simulink model "gm_Copy_of_uz_pmsm_model_9ph_21b_all_double_vnl"  (R2022a)
settings: Solver=FixedStepAuto  StartTime=0.0  StopTime=0.8  RelTol=1e-3
PreLoadFcn:
  | uz_pmsm_model_9ph_init_parameter
undefined symbols (not defined in the file or in its folder): a, b, c, friction_coefficient, inertia, k_i_d, k_i_q, k_p_d, k_p_q, Kpd, L_d, L_o1, L_o2, L_q, L_x1, L_x2, L_y1, L_y2, L_zero, polepair, psi_pm, R_1, static_friction_torque, Tnd, ts
libraries: hdlsllib x91, hdlmdlgenlib x21, simulink x18, slpidlib x2, spsAlphaBetaZerotodq0Lib x1, pid_lib x1, spsdq0toAlphaBetaZeroLib x1
(part 3 of 4)

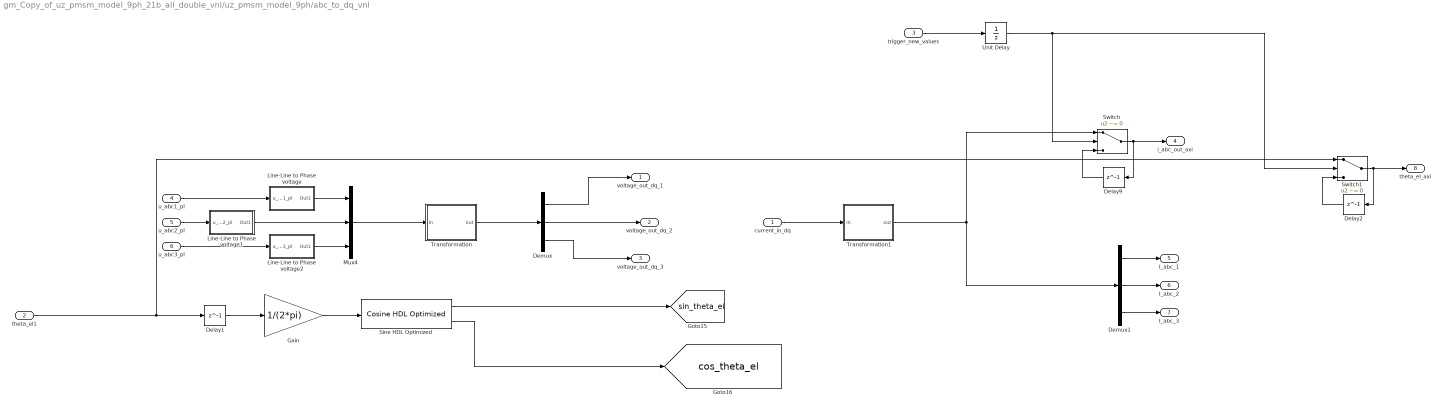
== system gm_Copy_of_uz_pmsm_model_9ph_21b_all_double_vnl/uz_pmsm_model_9ph/abc_to_dq_vnl ==
  current_in_dq : Inport
  theta_el1 : Inport  Port=2
  trigger_new_values : Inport  Port=3
  u_abc1_pl : Inport  Port=4
  u_abc2_pl : Inport  Port=5
  u_abc3_pl : Inport  Port=6
  Delay1 : Delay  DelayLength=1
  Delay2 : Delay  DelayLength=1
  Delay9 : Delay  DelayLength=1
  Demux : Demux  Outputs=3
  Demux1 : Demux  Outputs=3
  Gain : Gain  Gain=1/(2*pi)  OutDataTypeStr=fixdt(1,18,16)
  Line-Line to Phase voltage : Subsystem
  Line-Line to Phase voltage1 : Subsystem
  Line-Line to Phase voltage2 : Subsystem
  Mux4 : Mux  Inputs=3
  Sine HDL Optimized : hdlsllib/Lookup Tables/Cosine HDL Optimized  OutputFormula=sin(2*pi*u) and cos(2*pi*u)  NumDataPoints=64  TableDataTypeStr=fixdt(0,16,15)  SimulateLUTROMDelay=off
      settings: SourceProductBaseCode=SL
  Switch : Switch  Criteria=u2 ~= 0  SaturateOnIntegerOverflow=off  InputSameDT=off
  Switch1 : Switch  Criteria=u2 ~= 0  SaturateOnIntegerOverflow=off  InputSameDT=off
  Transformation : Subsystem
  Transformation1 : Subsystem
  Unit Delay : UnitDelay  SampleTime=-1  HasFrameUpgradeWarning=on
  voltage_out_dq_1 : Outport
  voltage_out_dq_2 : Outport  Port=2
  voltage_out_dq_3 : Outport  Port=3
  i_abc_out_axi : Outport  Port=4
  I_abc_1 : Outport  Port=5
  I_abc_2 : Outport  Port=6
  I_abc_3 : Outport  Port=7
  theta_el_axi : Outport  Port=8
  tag scope: cos_theta_el=global, sin_theta_el=global
  wires:
  Unit Delay/1 -> Switch/2, Switch1/2
  Switch1/1 -> Delay2/1, theta_el_axi/1
  Delay2/1 -> Switch1/3
  theta_el1/1 -> Switch1/1, Delay1/1
  Sine HDL Optimized/2 -> [cos_theta_el]
  Sine HDL Optimized/1 -> [sin_theta_el]
  Demux/3 -> voltage_out_dq_3/1
  Demux/2 -> voltage_out_dq_2/1
  Demux/1 -> voltage_out_dq_1/1
  Gain/1 -> Sine HDL Optimized/1
  u_abc1_pl/1 -> Line-Line to Phase voltage/1(u_abc1_pl)
  current_in_dq/1 -> Transformation1/1(in)
  Transformation/1(out) -> Demux/1
  Delay1/1 -> Gain/1
  Demux1/3 -> I_abc_3/1
  Switch/1 -> Delay9/1, i_abc_out_axi/1
  Demux1/1 -> I_abc_1/1
  u_abc3_pl/1 -> Line-Line to Phase voltage2/1(u_abc3_pl)
  trigger_new_values/1 -> Unit Delay/1
  Demux1/2 -> I_abc_2/1
  Mux4/1 -> Transformation/1(in)
  Delay9/1 -> Switch/3
  Line-Line to Phase voltage1/1(Out1) -> Mux4/2
  u_abc2_pl/1 -> Line-Line to Phase voltage1/1(u_abc2_pl)
  Line-Line to Phase voltage2/1(Out1) -> Mux4/3
  Line-Line to Phase voltage/1(Out1) -> Mux4/1
  Transformation1/1(out) -> Demux1/1, Switch/1

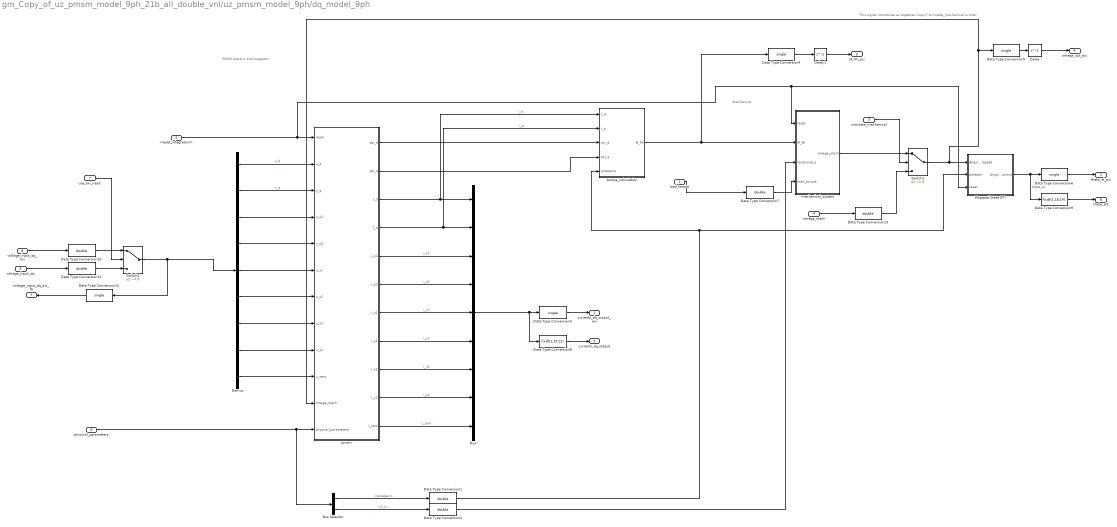
== system gm_Copy_of_uz_pmsm_model_9ph_21b_all_double_vnl/uz_pmsm_model_9ph/dq_model_9ph ==
  note: Mechanical
  note: PMSM electric and magentic
  note: This signal introduces an algebraic loop if simulate_mechanical is true!
  load_torque : Inport
  <reset_integrators> : Inport  Port=2
  simulate_mechanical : Inport  Port=3
  omega_mech : Inport  Port=4
  voltage_input_dq : Inport  Port=5
  physical_parameters : Inport  Port=6
  use_axi_input : Inport  Port=7
  voltage_input_dq_axi : Inport  Port=8
  Bus Selector : BusSelector  OutputSignals=polepair,1_J
  Data Type Conversion{1..2,7,10..11,13} (6 alike) : DataTypeConversion  OutDataTypeStr=double  RndMeth=Nearest  SaturateOnIntegerOverflow=off
  Data Type Conversion{3..6,12} (5 alike) : DataTypeConversion  OutDataTypeStr=single  RndMeth=Nearest  SaturateOnIntegerOverflow=off
  Data Type Conversion8 : DataTypeConversion  OutDataTypeStr=fixdt(1,25,12)  RndMeth=Nearest  SaturateOnIntegerOverflow=off
  Data Type Conversion9 : DataTypeConversion  OutDataTypeStr=fixdt(1,18,14)  RndMeth=Nearest  SaturateOnIntegerOverflow=off
  Delay : Delay  DelayLength=1
  Delay1 : Delay  DelayLength=1
  Demux : Demux  Outputs=9
  Mux : Mux  Inputs=9
  Switch1 : Switch  Criteria=u2 ~= 0  SaturateOnIntegerOverflow=off  InputSameDT=off
  Switch2 : Switch  Criteria=u2 ~= 0  SaturateOnIntegerOverflow=off  InputSameDT=off
  Wrapped State DTI : Subsystem
  mechanical_system : Subsystem
  pmsm : Subsystem
  torque_calculation : Subsystem
  currents_dq_output_axi : Outport
  theta_el_axi : Outport  Port=2
  M_Mi_axi : Outport  Port=3
  omega_out_axi : Outport  Port=4
  currents_dq_output : Outport  Port=5
  theta_el1 : Outport  Port=6
  voltage_input_dq_axi_fb : Outport  Port=7
  wires:
  Data Type Conversion13/1 -> Switch1/3
  Data Type Conversion12/1 -> voltage_input_dq_axi_fb/1
  Data Type Conversion11/1 -> Switch2/3
  Data Type Conversion10/1 -> Switch2/1
  voltage_input_dq_axi/1 -> Data Type Conversion10/1
  voltage_input_dq/1 -> Data Type Conversion11/1
  use_axi_input/1 -> Switch2/2
  Data Type Conversion9/1 -> theta_el1/1
  Data Type Conversion8/1 -> currents_dq_output/1
  Data Type Conversion7/1 -> mechanical_system/4(load_torque)
  Wrapped State DTI/1(Angular Position) -> Data Type Conversion6/1, Data Type Conversion9/1  "theta_el"
  Data Type Conversion6/1 -> theta_el_axi/1
  Data Type Conversion5/1 -> Delay/1
  Data Type Conversion4/1 -> Delay1/1
  Data Type Conversion3/1 -> currents_dq_output_axi/1
  Data Type Conversion2/1 -> mechanical_system/3(reciprocal_J)
  Data Type Conversion1/1 -> Wrapped State DTI/2(polepair), torque_calculation/5(polepairs)
  physical_parameters/1 -> pmsm/12(physical_parameters), Bus Selector/1
  Switch2/1 -> Demux/1, Data Type Conversion12/1
  Delay1/1 -> M_Mi_axi/1
  Delay/1 -> omega_out_axi/1
  Bus Selector/2 -> Data Type Conversion2/1  "<1_J>"
  Bus Selector/1 -> Data Type Conversion1/1  "<polepair>"
  Mux/1 -> Data Type Conversion3/1, Data Type Conversion8/1
  pmsm/8(i_y1) -> Mux/6  "i_y1"
  Switch1/1 -> Wrapped State DTI/1(Angular Speed), Data Type Conversion5/1, pmsm/11(omega_mech)
  load_torque/1 -> Data Type Conversion7/1
  mechanical_system/1(omega_mech) -> Switch1/1
  pmsm/4(I_q) -> Mux/2, torque_calculation/2(I_q)  "i_q"
  <reset_integrators>/1 -> pmsm/1(reset), mechanical_system/1(reset), Wrapped State DTI/3(reset)
  pmsm/5(i_o1) -> Mux/3  "i_o1"
  Demux/6 -> pmsm/7(u_y1)
  simulate_mechanical/1 -> Switch1/2
  pmsm/2(psi_q) -> torque_calculation/4(psi_q)
  omega_mech/1 -> Data Type Conversion13/1
  pmsm/1(psi_d) -> torque_calculation/3(psi_d)
  Demux/8 -> pmsm/9(u_y2)
  torque_calculation/1(M_Mi) -> mechanical_system/2(M_Mi), Data Type Conversion4/1
  pmsm/10(i_y2) -> Mux/8  "i_y2"
  pmsm/7(i_x1) -> Mux/5  "i_x1"
  pmsm/9(i_x2) -> Mux/7  "i_x2"
  Demux/9 -> pmsm/10(u_zero)
  Demux/2 -> pmsm/3(u_q)  "u_q"
  Demux/4 -> pmsm/5(u_o2)
  pmsm/6(i_o2) -> Mux/4  "i_o2"
  pmsm/11(i_zero) -> Mux/9  "i_zero"
  Demux/1 -> pmsm/2(u_d)  "u_d"
  pmsm/3(I_d) -> Mux/1, torque_calculation/1(I_d)  "i_d"
  Demux/3 -> pmsm/4(u_o1)
  Demux/7 -> pmsm/8(u_x2)
  Demux/5 -> pmsm/6(u_x1)

== system gm_Copy_of_uz_pmsm_model_9ph_21b_all_double_vnl/uz_pmsm_model_9ph/Compare/Assert_I_abc_1 ==
  cosim : Inport
  dut : Inport  Port=2
  AssertEq : Assertion  StopWhenAssertionFail=off
  Compare To Zero : simulink/Logic and Bit Operations/Compare To Zero  relop===  OutDataTypeStr=boolean
  Constant1 : Constant  Value=0  OutDataTypeStr=Inherit: Inherit via back propagation  SampleTime=-1
  Counter : simulink/Sources/Counter Free-Running  NumBits=32  tsamp=-1
  IgnoreCycles : Constant  Value=37  OutDataTypeStr=Inherit: Inherit via back propagation  SampleTime=-1
  Relational Operator : RelationalOperator  Operator=<  OutDataTypeStr=boolean  InputSameDT=off
  Relational Operator1 : RelationalOperator  Operator===  OutDataTypeStr=boolean  InputSameDT=off
  Switch : Switch  Criteria=u2 ~= 0  SaturateOnIntegerOverflow=off  InputSameDT=off
  Switch1 : Switch  Criteria=u2 ~= 0  SaturateOnIntegerOverflow=off  InputSameDT=off
  compare: I_abc_1 : Scope  NumInputPorts=3
  wires:
  Compare To Zero/1 -> compare: I_abc_1/3
  Relational Operator1/1 -> Compare To Zero/1, AssertEq/1  "err"
  Switch1/1 -> compare: I_abc_1/1, Relational Operator1/1
  Switch/1 -> compare: I_abc_1/2, Relational Operator1/2
  Constant1/1 -> Switch/1, Switch1/1
  Relational Operator/1 -> Switch/2, Switch1/2
  cosim/1 -> Switch1/3  "cosim"
  dut/1 -> Switch/3  "dut ref"
  Counter/1 -> Relational Operator/1
  IgnoreCycles/1 -> Relational Operator/2

== system gm_Copy_of_uz_pmsm_model_9ph_21b_all_double_vnl/uz_pmsm_model_9ph/Compare/Assert_I_abc_2 ==
  cosim : Inport
  dut : Inport  Port=2
  AssertEq : Assertion  StopWhenAssertionFail=off
  Compare To Zero : simulink/Logic and Bit Operations/Compare To Zero  relop===  OutDataTypeStr=boolean
  Constant1 : Constant  Value=0  OutDataTypeStr=Inherit: Inherit via back propagation  SampleTime=-1
  Counter : simulink/Sources/Counter Free-Running  NumBits=32  tsamp=-1
  IgnoreCycles : Constant  Value=37  OutDataTypeStr=Inherit: Inherit via back propagation  SampleTime=-1
  Relational Operator : RelationalOperator  Operator=<  OutDataTypeStr=boolean  InputSameDT=off
  Relational Operator1 : RelationalOperator  Operator===  OutDataTypeStr=boolean  InputSameDT=off
  Switch : Switch  Criteria=u2 ~= 0  SaturateOnIntegerOverflow=off  InputSameDT=off
  Switch1 : Switch  Criteria=u2 ~= 0  SaturateOnIntegerOverflow=off  InputSameDT=off
  compare: I_abc_2 : Scope  NumInputPorts=3
  wires:
  Compare To Zero/1 -> compare: I_abc_2/3
  Relational Operator1/1 -> Compare To Zero/1, AssertEq/1  "err"
  Switch1/1 -> compare: I_abc_2/1, Relational Operator1/1
  Switch/1 -> compare: I_abc_2/2, Relational Operator1/2
  Constant1/1 -> Switch/1, Switch1/1
  Relational Operator/1 -> Switch/2, Switch1/2
  cosim/1 -> Switch1/3  "cosim"
  dut/1 -> Switch/3  "dut ref"
  Counter/1 -> Relational Operator/1
  IgnoreCycles/1 -> Relational Operator/2

== system gm_Copy_of_uz_pmsm_model_9ph_21b_all_double_vnl/uz_pmsm_model_9ph/Compare/Assert_I_abc_3 ==
  cosim : Inport
  dut : Inport  Port=2
  AssertEq : Assertion  StopWhenAssertionFail=off
  Compare To Zero : simulink/Logic and Bit Operations/Compare To Zero  relop===  OutDataTypeStr=boolean
  Constant1 : Constant  Value=0  OutDataTypeStr=Inherit: Inherit via back propagation  SampleTime=-1
  Counter : simulink/Sources/Counter Free-Running  NumBits=32  tsamp=-1
  IgnoreCycles : Constant  Value=37  OutDataTypeStr=Inherit: Inherit via back propagation  SampleTime=-1
  Relational Operator : RelationalOperator  Operator=<  OutDataTypeStr=boolean  InputSameDT=off
  Relational Operator1 : RelationalOperator  Operator===  OutDataTypeStr=boolean  InputSameDT=off
  Switch : Switch  Criteria=u2 ~= 0  SaturateOnIntegerOverflow=off  InputSameDT=off
  Switch1 : Switch  Criteria=u2 ~= 0  SaturateOnIntegerOverflow=off  InputSameDT=off
  compare: I_abc_3 : Scope  NumInputPorts=3
  wires:
  Compare To Zero/1 -> compare: I_abc_3/3
  Relational Operator1/1 -> Compare To Zero/1, AssertEq/1  "err"
  Switch1/1 -> compare: I_abc_3/1, Relational Operator1/1
  Switch/1 -> compare: I_abc_3/2, Relational Operator1/2
  Constant1/1 -> Switch/1, Switch1/1
  Relational Operator/1 -> Switch/2, Switch1/2
  cosim/1 -> Switch1/3  "cosim"
  dut/1 -> Switch/3  "dut ref"
  Counter/1 -> Relational Operator/1
  IgnoreCycles/1 -> Relational Operator/2

== system gm_Copy_of_uz_pmsm_model_9ph_21b_all_double_vnl/uz_pmsm_model_9ph/Compare/Assert_i_abc_out_axi ==
  cosim : Inport
  dut : Inport  Port=2
  AssertEq : Assertion  StopWhenAssertionFail=off
  Compare To Zero : simulink/Logic and Bit Operations/Compare To Zero  relop===  OutDataTypeStr=boolean
  Constant1 : Constant  Value=0  OutDataTypeStr=Inherit: Inherit via back propagation  SampleTime=-1
  Counter : simulink/Sources/Counter Free-Running  NumBits=32  tsamp=-1
  IgnoreCycles : Constant  Value=37  OutDataTypeStr=Inherit: Inherit via back propagation  SampleTime=-1
  Relational Operator : RelationalOperator  Operator=<  OutDataTypeStr=boolean  InputSameDT=off
  Relational Operator1 : RelationalOperator  Operator===  OutDataTypeStr=boolean  InputSameDT=off
  Switch : Switch  Criteria=u2 ~= 0  SaturateOnIntegerOverflow=off  InputSameDT=off
  Switch1 : Switch  Criteria=u2 ~= 0  SaturateOnIntegerOverflow=off  InputSameDT=off
  compare: i_abc_out_axi : Scope  NumInputPorts=3
  wires:
  Compare To Zero/1 -> compare: i_abc_out_axi/3
  Relational Operator1/1 -> Compare To Zero/1, AssertEq/1  "err"
  Switch1/1 -> compare: i_abc_out_axi/1, Relational Operator1/1
  Switch/1 -> compare: i_abc_out_axi/2, Relational Operator1/2
  Constant1/1 -> Switch/1, Switch1/1
  Relational Operator/1 -> Switch/2, Switch1/2
  cosim/1 -> Switch1/3  "cosim"
  dut/1 -> Switch/3  "dut ref"
  Counter/1 -> Relational Operator/1
  IgnoreCycles/1 -> Relational Operator/2

== system gm_Copy_of_uz_pmsm_model_9ph_21b_all_double_vnl/uz_pmsm_model_9ph/Compare/Assert_theta_el_axi ==
  cosim : Inport
  dut : Inport  Port=2
  AssertEq : Assertion  StopWhenAssertionFail=off
  Compare To Zero : simulink/Logic and Bit Operations/Compare To Zero  relop===  OutDataTypeStr=boolean
  Constant1 : Constant  Value=0  OutDataTypeStr=Inherit: Inherit via back propagation  SampleTime=-1
  Counter : simulink/Sources/Counter Free-Running  NumBits=32  tsamp=-1
  IgnoreCycles : Constant  Value=37  OutDataTypeStr=Inherit: Inherit via back propagation  SampleTime=-1
  Relational Operator : RelationalOperator  Operator=<  OutDataTypeStr=boolean  InputSameDT=off
  Relational Operator1 : RelationalOperator  Operator===  OutDataTypeStr=boolean  InputSameDT=off
  Switch : Switch  Criteria=u2 ~= 0  SaturateOnIntegerOverflow=off  InputSameDT=off
  Switch1 : Switch  Criteria=u2 ~= 0  SaturateOnIntegerOverflow=off  InputSameDT=off
  compare: theta_el_axi : Scope  NumInputPorts=3
  wires:
  Compare To Zero/1 -> compare: theta_el_axi/3
  Relational Operator1/1 -> Compare To Zero/1, AssertEq/1  "err"
  Switch1/1 -> compare: theta_el_axi/1, Relational Operator1/1
  Switch/1 -> compare: theta_el_axi/2, Relational Operator1/2
  Constant1/1 -> Switch/1, Switch1/1
  Relational Operator/1 -> Switch/2, Switch1/2
  cosim/1 -> Switch1/3  "cosim"
  dut/1 -> Switch/3  "dut ref"
  Counter/1 -> Relational Operator/1
  IgnoreCycles/1 -> Relational Operator/2

== system gm_Copy_of_uz_pmsm_model_9ph_21b_all_double_vnl/uz_pmsm_model_9ph/Compare/Assert_voltage_out_dq_1 ==
  cosim : Inport
  dut : Inport  Port=2
  AssertEq : Assertion  StopWhenAssertionFail=off
  Compare To Zero : simulink/Logic and Bit Operations/Compare To Zero  relop===  OutDataTypeStr=boolean
  Constant1 : Constant  Value=0  OutDataTypeStr=Inherit: Inherit via back propagation  SampleTime=-1
  Counter : simulink/Sources/Counter Free-Running  NumBits=32  tsamp=-1
  IgnoreCycles : Constant  Value=37  OutDataTypeStr=Inherit: Inherit via back propagation  SampleTime=-1
  Relational Operator : RelationalOperator  Operator=<  OutDataTypeStr=boolean  InputSameDT=off
  Relational Operator1 : RelationalOperator  Operator===  OutDataTypeStr=boolean  InputSameDT=off
  Switch : Switch  Criteria=u2 ~= 0  SaturateOnIntegerOverflow=off  InputSameDT=off
  Switch1 : Switch  Criteria=u2 ~= 0  SaturateOnIntegerOverflow=off  InputSameDT=off
  compare: voltage_out_dq_1 : Scope  NumInputPorts=3
  wires:
  Compare To Zero/1 -> compare: voltage_out_dq_1/3
  Relational Operator1/1 -> Compare To Zero/1, AssertEq/1  "err"
  Switch1/1 -> compare: voltage_out_dq_1/1, Relational Operator1/1
  Switch/1 -> compare: voltage_out_dq_1/2, Relational Operator1/2
  Constant1/1 -> Switch/1, Switch1/1
  Relational Operator/1 -> Switch/2, Switch1/2
  cosim/1 -> Switch1/3  "cosim"
  dut/1 -> Switch/3  "dut ref"
  Counter/1 -> Relational Operator/1
  IgnoreCycles/1 -> Relational Operator/2

== system gm_Copy_of_uz_pmsm_model_9ph_21b_all_double_vnl/uz_pmsm_model_9ph/Compare/Assert_voltage_out_dq_2 ==
  cosim : Inport
  dut : Inport  Port=2
  AssertEq : Assertion  StopWhenAssertionFail=off
  Compare To Zero : simulink/Logic and Bit Operations/Compare To Zero  relop===  OutDataTypeStr=boolean
  Constant1 : Constant  Value=0  OutDataTypeStr=Inherit: Inherit via back propagation  SampleTime=-1
  Counter : simulink/Sources/Counter Free-Running  NumBits=32  tsamp=-1
  IgnoreCycles : Constant  Value=37  OutDataTypeStr=Inherit: Inherit via back propagation  SampleTime=-1
  Relational Operator : RelationalOperator  Operator=<  OutDataTypeStr=boolean  InputSameDT=off
  Relational Operator1 : RelationalOperator  Operator===  OutDataTypeStr=boolean  InputSameDT=off
  Switch : Switch  Criteria=u2 ~= 0  SaturateOnIntegerOverflow=off  InputSameDT=off
  Switch1 : Switch  Criteria=u2 ~= 0  SaturateOnIntegerOverflow=off  InputSameDT=off
  compare: voltage_out_dq_2 : Scope  NumInputPorts=3
  wires:
  Compare To Zero/1 -> compare: voltage_out_dq_2/3
  Relational Operator1/1 -> Compare To Zero/1, AssertEq/1  "err"
  Switch1/1 -> compare: voltage_out_dq_2/1, Relational Operator1/1
  Switch/1 -> compare: voltage_out_dq_2/2, Relational Operator1/2
  Constant1/1 -> Switch/1, Switch1/1
  Relational Operator/1 -> Switch/2, Switch1/2
  cosim/1 -> Switch1/3  "cosim"
  dut/1 -> Switch/3  "dut ref"
  Counter/1 -> Relational Operator/1
  IgnoreCycles/1 -> Relational Operator/2

== system gm_Copy_of_uz_pmsm_model_9ph_21b_all_double_vnl/uz_pmsm_model_9ph/Compare/Assert_voltage_out_dq_3 ==
  cosim : Inport
  dut : Inport  Port=2
  AssertEq : Assertion  StopWhenAssertionFail=off
  Compare To Zero : simulink/Logic and Bit Operations/Compare To Zero  relop===  OutDataTypeStr=boolean
  Constant1 : Constant  Value=0  OutDataTypeStr=Inherit: Inherit via back propagation  SampleTime=-1
  Counter : simulink/Sources/Counter Free-Running  NumBits=32  tsamp=-1
  IgnoreCycles : Constant  Value=37  OutDataTypeStr=Inherit: Inherit via back propagation  SampleTime=-1
  Relational Operator : RelationalOperator  Operator=<  OutDataTypeStr=boolean  InputSameDT=off
  Relational Operator1 : RelationalOperator  Operator===  OutDataTypeStr=boolean  InputSameDT=off
  Switch : Switch  Criteria=u2 ~= 0  SaturateOnIntegerOverflow=off  InputSameDT=off
  Switch1 : Switch  Criteria=u2 ~= 0  SaturateOnIntegerOverflow=off  InputSameDT=off
  compare: voltage_out_dq_3 : Scope  NumInputPorts=3
  wires:
  Compare To Zero/1 -> compare: voltage_out_dq_3/3
  Relational Operator1/1 -> Compare To Zero/1, AssertEq/1  "err"
  Switch1/1 -> compare: voltage_out_dq_3/1, Relational Operator1/1
  Switch/1 -> compare: voltage_out_dq_3/2, Relational Operator1/2
  Constant1/1 -> Switch/1, Switch1/1
  Relational Operator/1 -> Switch/2, Switch1/2
  cosim/1 -> Switch1/3  "cosim"
  dut/1 -> Switch/3  "dut ref"
  Counter/1 -> Relational Operator/1
  IgnoreCycles/1 -> Relational Operator/2

== system gm_Copy_of_uz_pmsm_model_9ph_21b_all_double_vnl/uz_pmsm_model_9ph/Compare/CleanupScopes ==

== system gm_Copy_of_uz_pmsm_model_9ph_21b_all_double_vnl/uz_pmsm_model_9ph/Compare/Enable ==

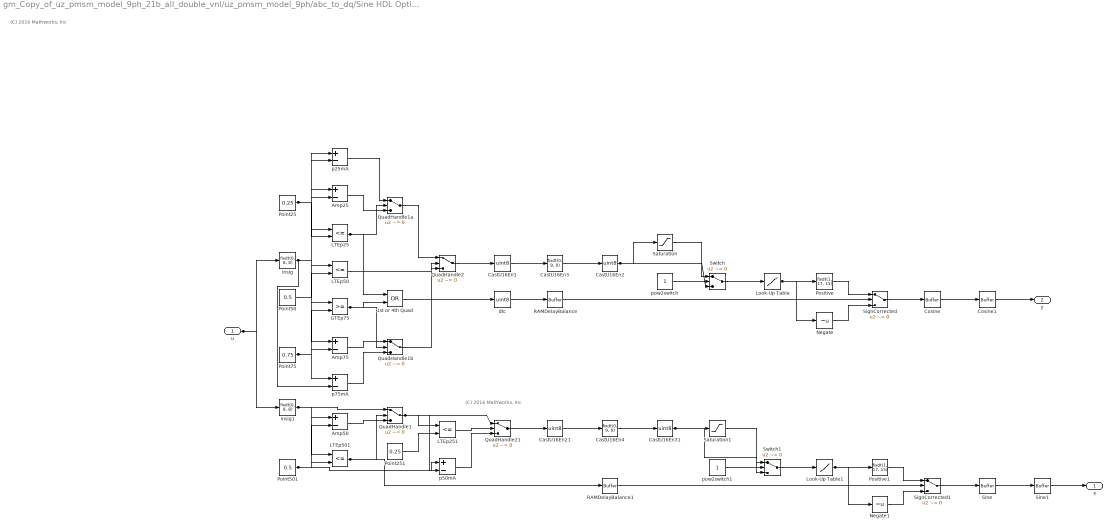
== system gm_Copy_of_uz_pmsm_model_9ph_21b_all_double_vnl/uz_pmsm_model_9ph/abc_to_dq/Sine HDL Optimized ==
  note: (C) 2016 Mathworks, Inc
  note: (C) 2016 Mathworks, Inc
  u : Inport  OutDataTypeStr=fixdt(1,18,16,'DataTypeOverride', 'Off')  SampleTime=1e-08
  1st or 4th Quad : Logic  Operator=OR  AllPortsSameDT=off  OutDataTypeStr=boolean  SampleTime=1e-08
  Amp25 : Sum  Inputs=+-  AccumDataTypeStr=fixdt(1, 18, 17)  OutDataTypeStr=fixdt(1, 18, 17)  SampleTime=1e-08
  Amp50 : Sum  Inputs=+-  AccumDataTypeStr=fixdt(1, 18, 17)  OutDataTypeStr=fixdt(1, 18, 17)  SampleTime=1e-08
  Amp75 : Sum  Inputs=+-  AccumDataTypeStr=fixdt(1, 18, 17)  OutDataTypeStr=fixdt(1, 18, 17)  SampleTime=1e-08
  CastU16En1 : DataTypeConversion  OutDataTypeStr=uint8  ConvertRealWorld=Stored Integer (SI)  SampleTime=1e-08  SaturateOnIntegerOverflow=off  RndMeth=Floor
  CastU16En2 : DataTypeConversion  OutDataTypeStr=uint8  ConvertRealWorld=Stored Integer (SI)  SampleTime=1e-08  RndMeth=Floor
  CastU16En21 : DataTypeConversion  OutDataTypeStr=uint8  ConvertRealWorld=Stored Integer (SI)  SampleTime=1e-08  SaturateOnIntegerOverflow=off  RndMeth=Floor
  CastU16En3 : DataTypeConversion  OutDataTypeStr=fixdt(0, 9, 0)  SampleTime=1e-08  SaturateOnIntegerOverflow=off  RndMeth=Floor
  CastU16En31 : DataTypeConversion  OutDataTypeStr=uint8  ConvertRealWorld=Stored Integer (SI)  SampleTime=1e-08  RndMeth=Floor
  CastU16En4 : DataTypeConversion  OutDataTypeStr=fixdt(0, 9, 0)  SampleTime=1e-08  SaturateOnIntegerOverflow=off  RndMeth=Floor
  Cosine : hdlmdlgenlib/Buffer
      settings: SourceProductBaseCode=SL
  Cosine1 : hdlmdlgenlib/Buffer
      settings: SourceProductBaseCode=SL
  GTEp75 : RelationalOperator  OutDataTypeStr=boolean  SampleTime=1e-08  InputSameDT=off
  LTEp{25,50,251,501} (4 alike) : RelationalOperator  Operator=<=  OutDataTypeStr=boolean  SampleTime=1e-08  InputSameDT=off
  Look-Up Table : Lookup_n-D  NumberOfTableDimensions=1  BreakpointsForDimension1="fi(\"numerictype\",numerictype(0,8,0),\"fimath\",fimath(\"RoundingMethod\", \"Floor\",\"OverflowAction\", \"Wrap\",\"ProductMode\",\"FullPrecision\",\"SumMode\",\"FullPrecision\"),\"Value\",\"[0 1 2 3 4 5 6 7 8 9 10 11 12 13 14 15 16 17 18 19 20 21 22 23 24 25 26 27 28 29 30 31 32 33 34 35 36 37 38 39 40 41 42 43 44 45 46 47 48 49 50 51 52 53 54 55 56 57 58 59 60 61 62 63]\")"  Table="reshape(fi(\"numerictype\",numerictype(1,17,15),\"fimath\",fimath(\"RoundingMethod\", \"Floor\",\"OverflowAction\", \"Wrap\",\"ProductMode\",\"FullPrecision\",\"SumMode\",\"FullPrecision\"),\"Value\",\"[0;0.0245361328125;0.049072265625;0.073577880859375;0.0980224609375;0.122406005859375;0.146728515625;0.17095947265625;0.195098876953125;0.2191162109375;0.24298095703125;0.2667236328125;0.290283203125;0.313690185546875;0.336883544921875;0.359893798828125;0.3826904296875;0.405242919921875;0.42755126953125;0.449615478515625;0.471405029296875;0.492889404296875;0.51409912109375;0.535003662109375;0.555572509765625;0.5758056640625;0.595703125;0.615234375;0.6343994140625;0.653167724609375;0.67156982421875;0.689544677734375;0.70709228515625;0.7242431640625;0.740936279296875;0.7572021484375;0.77301025390625;0.788360595703125;0.80322265625;0.817596435546875;0.83148193359375;0.8448486328125;0.85772705078125;0.870086669921875;0.881927490234375;0.893218994140625;0.90399169921875;0.914215087890625;0.92388916015625;0.9329833984375;0.941558837890625;0.94952392578125;0.956939697265625;0.963775634765625;0.97003173828125;0.9757080078125;0.98077392578125;0.98529052734375;0.989166259765625;0.99249267578125;0.99517822265625;0.997283935546875;0.998809814453125;0.99969482421875]\"), [1  64])"  InterpMethod=Flat  ExtrapMethod=Clip  DiagnosticForOutOfRangeInput=Error  SampleTime=1e-08  OutDataTypeStr=fixdt(1, 17, 15)
  Look-Up Table1 : Lookup_n-D  NumberOfTableDimensions=1  BreakpointsForDimension1="fi(\"numerictype\",numerictype(0,8,0),\"fimath\",fimath(\"RoundingMethod\", \"Floor\",\"OverflowAction\", \"Wrap\",\"ProductMode\",\"FullPrecision\",\"SumMode\",\"FullPrecision\"),\"Value\",\"[0 1 2 3 4 5 6 7 8 9 10 11 12 13 14 15 16 17 18 19 20 21 22 23 24 25 26 27 28 29 30 31 32 33 34 35 36 37 38 39 40 41 42 43 44 45 46 47 48 49 50 51 52 53 54 55 56 57 58 59 60 61 62 63]\")"  Table="reshape(fi(\"numerictype\",numerictype(1,17,15),\"fimath\",fimath(\"RoundingMethod\", \"Floor\",\"OverflowAction\", \"Wrap\",\"ProductMode\",\"FullPrecision\",\"SumMode\",\"FullPrecision\"),\"Value\",\"[0;0.0245361328125;0.049072265625;0.073577880859375;0.0980224609375;0.122406005859375;0.146728515625;0.17095947265625;0.195098876953125;0.2191162109375;0.24298095703125;0.2667236328125;0.290283203125;0.313690185546875;0.336883544921875;0.359893798828125;0.3826904296875;0.405242919921875;0.42755126953125;0.449615478515625;0.471405029296875;0.492889404296875;0.51409912109375;0.535003662109375;0.555572509765625;0.5758056640625;0.595703125;0.615234375;0.6343994140625;0.653167724609375;0.67156982421875;0.689544677734375;0.70709228515625;0.7242431640625;0.740936279296875;0.7572021484375;0.77301025390625;0.788360595703125;0.80322265625;0.817596435546875;0.83148193359375;0.8448486328125;0.85772705078125;0.870086669921875;0.881927490234375;0.893218994140625;0.90399169921875;0.914215087890625;0.92388916015625;0.9329833984375;0.941558837890625;0.94952392578125;0.956939697265625;0.963775634765625;0.97003173828125;0.9757080078125;0.98077392578125;0.98529052734375;0.989166259765625;0.99249267578125;0.99517822265625;0.997283935546875;0.998809814453125;0.99969482421875]\"), [1  64])"  InterpMethod=Flat  ExtrapMethod=Clip  DiagnosticForOutOfRangeInput=Error  SampleTime=1e-08  OutDataTypeStr=fixdt(1, 17, 15)
  Negate : UnaryMinus  SampleTime=1e-08
  Negate1 : UnaryMinus  SampleTime=1e-08
  Point25 : Constant  Value=0.25  OutDataTypeStr=fixdt(0, 17, 17)  SampleTime=1e-08
  Point251 : Constant  Value=0.25  OutDataTypeStr=fixdt(0, 17, 17)  SampleTime=1e-08
  Point50 : Constant  Value=0.5  OutDataTypeStr=fixdt(0, 17, 17)  SampleTime=1e-08
  Point501 : Constant  Value=0.5  OutDataTypeStr=fixdt(0, 17, 17)  SampleTime=1e-08
  Point75 : Constant  Value=0.75  OutDataTypeStr=fixdt(0, 17, 17)  SampleTime=1e-08
  Positive : DataTypeConversion  OutDataTypeStr=fixdt(1, 17, 15)  SampleTime=1e-08  SaturateOnIntegerOverflow=off  RndMeth=Floor
  Positive1 : DataTypeConversion  OutDataTypeStr=fixdt(1, 17, 15)  SampleTime=1e-08  SaturateOnIntegerOverflow=off  RndMeth=Floor
  QuadHandle1 : Switch  Criteria=u2 ~= 0  Threshold=double(0)  OutDataTypeStr=fixdt(1, 18, 17)  SampleTime=1e-08  SaturateOnIntegerOverflow=off  InputSameDT=off
  QuadHandle1a : Switch  Criteria=u2 ~= 0  Threshold=double(0)  OutDataTypeStr=fixdt(1, 18, 17)  SampleTime=1e-08  SaturateOnIntegerOverflow=off  InputSameDT=off
  QuadHandle1b : Switch  Criteria=u2 ~= 0  Threshold=double(0)  OutDataTypeStr=fixdt(1, 18, 17)  SampleTime=1e-08  SaturateOnIntegerOverflow=off  InputSameDT=off
  QuadHandle2 : Switch  Criteria=u2 ~= 0  Threshold=double(0)  OutDataTypeStr=fixdt(0, 8, 8)  SampleTime=1e-08  InputSameDT=off
  QuadHandle21 : Switch  Criteria=u2 ~= 0  Threshold=double(0)  OutDataTypeStr=fixdt(0, 8, 8)  SampleTime=1e-08  SaturateOnIntegerOverflow=off  InputSameDT=off
  RAMDelayBalance : hdlmdlgenlib/Buffer
      settings: SourceProductBaseCode=SL
  RAMDelayBalance1 : hdlmdlgenlib/Buffer
      settings: SourceProductBaseCode=SL
  Saturation : Saturate  UpperLimit="fi(0,0,8,0,\"hex\",\"3f\")"  LowerLimit="fi(0,0,8,0,\"hex\",\"00\")"  SampleTime=1e-08  OutDataTypeStr=uint8
  Saturation1 : Saturate  UpperLimit="fi(0,0,8,0,\"hex\",\"3f\")"  LowerLimit="fi(0,0,8,0,\"hex\",\"00\")"  SampleTime=1e-08  OutDataTypeStr=uint8
  SignCorrected : Switch  Criteria=u2 ~= 0  Threshold=double(0)  OutDataTypeStr=fixdt(1, 17, 15)  SampleTime=1e-08  SaturateOnIntegerOverflow=off  InputSameDT=off
  SignCorrected1 : Switch  Criteria=u2 ~= 0  Threshold=double(0)  OutDataTypeStr=fixdt(1, 17, 15)  SampleTime=1e-08  SaturateOnIntegerOverflow=off  InputSameDT=off
  Sine : hdlmdlgenlib/Buffer
      settings: SourceProductBaseCode=SL
  Sine1 : hdlmdlgenlib/Buffer
      settings: SourceProductBaseCode=SL
  Switch : Switch  Criteria=u2 ~= 0  Threshold=double(0)  OutDataTypeStr=uint8  SampleTime=1e-08  SaturateOnIntegerOverflow=off  InputSameDT=off
  Switch1 : Switch  Criteria=u2 ~= 0  Threshold=double(0)  OutDataTypeStr=uint8  SampleTime=1e-08  SaturateOnIntegerOverflow=off  InputSameDT=off
  dtc : DataTypeConversion  OutDataTypeStr=uint8  SampleTime=1e-08  SaturateOnIntegerOverflow=off  RndMeth=Floor
  insig : DataTypeConversion  OutDataTypeStr=fixdt(0, 8, 8)  SampleTime=1e-08  SaturateOnIntegerOverflow=off  RndMeth=Floor
  insig1 : DataTypeConversion  OutDataTypeStr=fixdt(0, 8, 8)  SampleTime=1e-08  SaturateOnIntegerOverflow=off  RndMeth=Floor
  p25mA : Sum  Inputs=+-  AccumDataTypeStr=fixdt(1, 18, 17)  OutDataTypeStr=fixdt(1, 18, 17)  SampleTime=1e-08
  p50mA : Sum  Inputs=+-  AccumDataTypeStr=fixdt(1, 19, 17)  OutDataTypeStr=fixdt(1, 19, 17)  SampleTime=1e-08
  p75mA : Sum  Inputs=+-  AccumDataTypeStr=fixdt(1, 18, 17)  OutDataTypeStr=fixdt(1, 18, 17)  SampleTime=1e-08
  pow2switch : Constant  OutDataTypeStr=boolean  SampleTime=1e-08
  pow2switch1 : Constant  OutDataTypeStr=boolean  SampleTime=1e-08
  x : Outport  SampleTime=1e-08
  y : Outport  Port=2  SampleTime=1e-08
  wires:
  u/1 -> insig/1, insig1/1
  1st or 4th Quad/1 -> dtc/1
  pow2switch1/1 -> Switch1/2
  p50mA/1 -> QuadHandle21/3
  insig1/1 -> Amp50/1, LTEp501/1, QuadHandle1/1
  Switch1/1 -> Look-Up Table1/1
  SignCorrected1/1 -> Sine/1
  Saturation1/1 -> Switch1/1
  RAMDelayBalance1/1 -> SignCorrected1/2
  QuadHandle21/1 -> CastU16En21/1
  QuadHandle1/1 -> LTEp251/1, QuadHandle21/1, p50mA/2
  Positive1/1 -> SignCorrected1/1
  Point501/1 -> Amp50/2, LTEp501/2, p50mA/1
  Point251/1 -> LTEp251/2
  Negate1/1 -> SignCorrected1/3
  Look-Up Table1/1 -> Negate1/1, Positive1/1
  LTEp501/1 -> RAMDelayBalance1/1, QuadHandle1/2
  LTEp251/1 -> QuadHandle21/2
  CastU16En4/1 -> CastU16En31/1
  CastU16En31/1 -> Saturation1/1, Switch1/3
  CastU16En21/1 -> CastU16En4/1
  Amp50/1 -> QuadHandle1/3
  pow2switch/1 -> Switch/2
  p75mA/1 -> QuadHandle1b/3
  p25mA/1 -> QuadHandle1a/1
  insig/1 -> Amp25/1, Amp75/1, GTEp75/1, LTEp25/1, LTEp50/1, p25mA/2, p75mA/2
  Switch/1 -> Look-Up Table/1
  SignCorrected/1 -> Cosine/1
  Saturation/1 -> Switch/1
  RAMDelayBalance/1 -> SignCorrected/2
  QuadHandle2/1 -> CastU16En1/1
  QuadHandle1b/1 -> QuadHandle2/3
  QuadHandle1a/1 -> QuadHandle2/1
  Positive/1 -> SignCorrected/1
  Point75/1 -> Amp75/2, GTEp75/2, p75mA/1
  Point50/1 -> LTEp50/2
  Point25/1 -> Amp25/2, LTEp25/2, p25mA/1
  Negate/1 -> SignCorrected/3
  Look-Up Table/1 -> Negate/1, Positive/1
  LTEp50/1 -> QuadHandle2/2
  LTEp25/1 -> 1st or 4th Quad/1, QuadHandle1a/2
  GTEp75/1 -> 1st or 4th Quad/2, QuadHandle1b/2
  CastU16En3/1 -> CastU16En2/1
  CastU16En2/1 -> Saturation/1, Switch/3
  CastU16En1/1 -> CastU16En3/1
  Amp75/1 -> QuadHandle1b/1
  Amp25/1 -> QuadHandle1a/3
  dtc/1 -> RAMDelayBalance/1
  Sine/1 -> Sine1/1
  Cosine/1 -> Cosine1/1
  Cosine1/1 -> y/1
  Sine1/1 -> x/1

== system gm_Copy_of_uz_pmsm_model_9ph_21b_all_double_vnl/uz_pmsm_model_9ph/abc_to_dq/t19 ==
  in0 : Inport
  ColVec1 : Selector  NumberOfDimensions=2  IndexOptions=Select all,Index vector (dialog)  Indices=1,1  OutputSizes=1,1
  ColVec2 : Selector  NumberOfDimensions=2  IndexOptions=Select all,Index vector (dialog)  Indices=1,2  OutputSizes=1,1
  ColVec3 : Selector  NumberOfDimensions=2  IndexOptions=Select all,Index vector (dialog)  Indices=1,3  OutputSizes=1,1
  ColVec4 : Selector  NumberOfDimensions=2  IndexOptions=Select all,Index vector (dialog)  Indices=1,4  OutputSizes=1,1
  ColVec5 : Selector  NumberOfDimensions=2  IndexOptions=Select all,Index vector (dialog)  Indices=1,5  OutputSizes=1,1
  ColVec6 : Selector  NumberOfDimensions=2  IndexOptions=Select all,Index vector (dialog)  Indices=1,6  OutputSizes=1,1
  ColVec7 : Selector  NumberOfDimensions=2  IndexOptions=Select all,Index vector (dialog)  Indices=1,7  OutputSizes=1,1
  ColVec8 : Selector  NumberOfDimensions=2  IndexOptions=Select all,Index vector (dialog)  Indices=1,8  OutputSizes=1,1
  ColVec9 : Selector  NumberOfDimensions=2  IndexOptions=Select all,Index vector (dialog)  Indices=1,9  OutputSizes=1,1
  out0 : Outport
  out1 : Outport  Port=2
  out2 : Outport  Port=3
  out3 : Outport  Port=4
  out4 : Outport  Port=5
  out5 : Outport  Port=6
  out6 : Outport  Port=7
  out7 : Outport  Port=8
  out8 : Outport  Port=9
  wires:
  ColVec9/1 -> out8/1
  ColVec8/1 -> out7/1
  ColVec7/1 -> out6/1
  ColVec6/1 -> out5/1
  ColVec5/1 -> out4/1
  ColVec4/1 -> out3/1
  ColVec3/1 -> out2/1
  ColVec2/1 -> out1/1
  ColVec1/1 -> out0/1
  in0/1 -> ColVec9/1, ColVec8/1, ColVec7/1, ColVec6/1, ColVec5/1, ColVec4/1, ColVec3/1, ColVec2/1, ColVec1/1

== system gm_Copy_of_uz_pmsm_model_9ph_21b_all_double_vnl/uz_pmsm_model_9ph/abc_to_dq/t23 ==
  in0 : Inport
  ColVec1 : Selector  NumberOfDimensions=2  IndexOptions=Select all,Index vector (dialog)  Indices=1,1  OutputSizes=1,1
  ColVec2 : Selector  NumberOfDimensions=2  IndexOptions=Select all,Index vector (dialog)  Indices=1,2  OutputSizes=1,1
  ColVec3 : Selector  NumberOfDimensions=2  IndexOptions=Select all,Index vector (dialog)  Indices=1,3  OutputSizes=1,1
  ColVec4 : Selector  NumberOfDimensions=2  IndexOptions=Select all,Index vector (dialog)  Indices=1,4  OutputSizes=1,1
  ColVec5 : Selector  NumberOfDimensions=2  IndexOptions=Select all,Index vector (dialog)  Indices=1,5  OutputSizes=1,1
  ColVec6 : Selector  NumberOfDimensions=2  IndexOptions=Select all,Index vector (dialog)  Indices=1,6  OutputSizes=1,1
  ColVec7 : Selector  NumberOfDimensions=2  IndexOptions=Select all,Index vector (dialog)  Indices=1,7  OutputSizes=1,1
  ColVec8 : Selector  NumberOfDimensions=2  IndexOptions=Select all,Index vector (dialog)  Indices=1,8  OutputSizes=1,1
  ColVec9 : Selector  NumberOfDimensions=2  IndexOptions=Select all,Index vector (dialog)  Indices=1,9  OutputSizes=1,1
  out0 : Outport
  out1 : Outport  Port=2
  out2 : Outport  Port=3
  out3 : Outport  Port=4
  out4 : Outport  Port=5
  out5 : Outport  Port=6
  out6 : Outport  Port=7
  out7 : Outport  Port=8
  out8 : Outport  Port=9
  wires:
  ColVec9/1 -> out8/1
  ColVec8/1 -> out7/1
  ColVec7/1 -> out6/1
  ColVec6/1 -> out5/1
  ColVec5/1 -> out4/1
  ColVec4/1 -> out3/1
  ColVec3/1 -> out2/1
  ColVec2/1 -> out1/1
  ColVec1/1 -> out0/1
  in0/1 -> ColVec9/1, ColVec8/1, ColVec7/1, ColVec6/1, ColVec5/1, ColVec4/1, ColVec3/1, ColVec2/1, ColVec1/1

== system gm_Copy_of_uz_pmsm_model_9ph_21b_all_double_vnl/uz_pmsm_model_9ph/abc_to_dq_vnl/Line-Line to Phase voltage ==
  u_abc1_pl : Inport
  Complex to Real-Imag : ComplexToRealImag
  Constant : Constant  Value=0  OutDataTypeStr=fixdt(1,25,12)  SampleTime=-1
  Constant1 : Constant  Value=1/sqrt(3)*exp(1i*-30/180*pi)  OutDataTypeStr=fixdt(1,18,16)  SampleTime=-1
  Demux3 : Demux  Outputs=3
  Mux4 : Mux  Inputs=3
  Product : Product  OutDataTypeStr=fixdt(1,25,12)
  Real-Imag to Complex : RealImagToComplex
  Terminator : Terminator
  abc   to   alpha_beta_0 : Subsystem
  alpha_beta_0   to   abc : Subsystem
  Out1 : Outport
  wires:
  Constant1/1 -> Product/2
  alpha_beta_0   to   abc/1("a, b, c") -> Out1/1
  abc   to   alpha_beta_0/1("alpha, beta, 0 ") -> Demux3/1
  Demux3/3 -> Terminator/1
  u_abc1_pl/1 -> abc   to   alpha_beta_0/1("a, b, c")
  Constant/1 -> Mux4/3
  Complex to Real-Imag/2 -> Mux4/2
  Demux3/1 -> Real-Imag to Complex/1
  Real-Imag to Complex/1 -> Product/1
  Product/1 -> Complex to Real-Imag/1
  Mux4/1 -> alpha_beta_0   to   abc/1("alpha, beta, 0  ")
  Complex to Real-Imag/1 -> Mux4/1
  Demux3/2 -> Real-Imag to Complex/2

== system gm_Copy_of_uz_pmsm_model_9ph_21b_all_double_vnl/uz_pmsm_model_9ph/abc_to_dq_vnl/Line-Line to Phase voltage1 ==
  u_abc2_pl : Inport
  Complex to Real-Imag : ComplexToRealImag
  Constant : Constant  Value=0  OutDataTypeStr=fixdt(1,25,12)  SampleTime=-1
  Constant1 : Constant  Value=1/sqrt(3)*exp(1i*-30/180*pi)  OutDataTypeStr=fixdt(1,18,16)  SampleTime=-1
  Demux3 : Demux  Outputs=3
  Mux4 : Mux  Inputs=3
  Product : Product  OutDataTypeStr=fixdt(1,25,12)
  Real-Imag to Complex : RealImagToComplex
  Terminator : Terminator
  abc   to   alpha_beta_0 : Subsystem
  alpha_beta_0   to   abc : Subsystem
  Out1 : Outport
  wires:
  Demux3/2 -> Real-Imag to Complex/2
  Complex to Real-Imag/1 -> Mux4/1
  Mux4/1 -> alpha_beta_0   to   abc/1("alpha, beta, 0  ")
  Product/1 -> Complex to Real-Imag/1
  Real-Imag to Complex/1 -> Product/1
  Demux3/1 -> Real-Imag to Complex/1
  Complex to Real-Imag/2 -> Mux4/2
  Constant/1 -> Mux4/3
  u_abc2_pl/1 -> abc   to   alpha_beta_0/1("a, b, c")
  Demux3/3 -> Terminator/1
  abc   to   alpha_beta_0/1("alpha, beta, 0 ") -> Demux3/1
  alpha_beta_0   to   abc/1("a, b, c") -> Out1/1
  Constant1/1 -> Product/2

== system gm_Copy_of_uz_pmsm_model_9ph_21b_all_double_vnl/uz_pmsm_model_9ph/abc_to_dq_vnl/Line-Line to Phase voltage2 ==
  u_abc3_pl : Inport
  Complex to Real-Imag : ComplexToRealImag
  Constant : Constant  Value=0  OutDataTypeStr=fixdt(1,25,12)  SampleTime=-1
  Constant1 : Constant  Value=1/sqrt(3)*exp(1i*-30/180*pi)  OutDataTypeStr=fixdt(1,18,16)  SampleTime=-1
  Demux3 : Demux  Outputs=3
  Mux4 : Mux  Inputs=3
  Product : Product  OutDataTypeStr=fixdt(1,25,12)
  Real-Imag to Complex : RealImagToComplex
  Terminator : Terminator
  abc   to   alpha_beta_0 : Subsystem
  alpha_beta_0   to   abc : Subsystem
  Out1 : Outport
  wires:
  Constant1/1 -> Product/2
  alpha_beta_0   to   abc/1("a, b, c") -> Out1/1
  abc   to   alpha_beta_0/1("alpha, beta, 0 ") -> Demux3/1
  Demux3/3 -> Terminator/1
  u_abc3_pl/1 -> abc   to   alpha_beta_0/1("a, b, c")
  Constant/1 -> Mux4/3
  Complex to Real-Imag/2 -> Mux4/2
  Demux3/1 -> Real-Imag to Complex/1
  Real-Imag to Complex/1 -> Product/1
  Product/1 -> Complex to Real-Imag/1
  Mux4/1 -> alpha_beta_0   to   abc/1("alpha, beta, 0  ")
  Complex to Real-Imag/1 -> Mux4/1
  Demux3/2 -> Real-Imag to Complex/2

== system gm_Copy_of_uz_pmsm_model_9ph_21b_all_double_vnl/uz_pmsm_model_9ph/abc_to_dq_vnl/Transformation ==
  in : Inport
  Add : Sum  OutDataTypeStr=fixdt(1,25,12)
  Add1 : Sum  Inputs=-+  OutDataTypeStr=fixdt(1,25,12)
  Constant1 : Constant  Value=c  OutDataTypeStr=fixdt(1,18,17)  SampleTime=-1
  Demux1 : Demux  Outputs=9
  Divide{,1..3} (4 alike) : Product  Inputs=**  OutDataTypeStr=fixdt(1,25,12)
  MatrixMultiply : Product  Multiplication=Matrix(*)  OutDataTypeStr=fixdt(1,25,12)
  Mux : Mux  Inputs=9
  out : Outport
  wires:
  in/1 -> MatrixMultiply/2
  MatrixMultiply/1 -> Demux1/1
  Constant1/1 -> MatrixMultiply/1
  Divide2/1 -> Add1/1
  Divide3/1 -> Add1/2
  [cos_theta_el] -> Divide3/1
  [sin_theta_el] -> Divide2/1
  [cos_theta_el] -> Divide/1  "cos_theta_hdl"
  [sin_theta_el] -> Divide1/1  "sin_theta_hdl"
  Divide1/1 -> Add/2
  Divide/1 -> Add/1
  Demux1/2 -> Divide3/2, Divide1/2  "u_beta"
  Demux1/1 -> Divide2/2, Divide/2  "u_alpha"
  Add/1 -> Mux/1
  Add1/1 -> Mux/2
  Mux/1 -> out/1  "trafo_out"
  Demux1/9 -> Mux/9
  Demux1/8 -> Mux/8
  Demux1/7 -> Mux/7
  Demux1/6 -> Mux/6
  Demux1/5 -> Mux/5
  Demux1/4 -> Mux/4
  Demux1/3 -> Mux/3

== system gm_Copy_of_uz_pmsm_model_9ph_21b_all_double_vnl/uz_pmsm_model_9ph/abc_to_dq_vnl/Transformation1 ==
  in : Inport
  Add : Sum  Inputs=+-  OutDataTypeStr=fixdt(1,25,12)
  Add1 : Sum  OutDataTypeStr=fixdt(1,25,12)
  Constant1 : Constant  Value=inv(c)  OutDataTypeStr=fixdt(1,18,16)  SampleTime=-1
  Data Type Conversion28 : DataTypeConversion  OutDataTypeStr=fixdt(1,25,12)  RndMeth=Nearest  SaturateOnIntegerOverflow=off
  Demux1 : Demux  Outputs=9
  Divide{,1..3} (4 alike) : Product  Inputs=**  OutDataTypeStr=fixdt(1,25,12)
  MatrixMultiply : Product  Multiplication=Matrix(*)  OutDataTypeStr=fixdt(1,25,12)
  Mux : Mux  Inputs=9
  out : Outport
  wires:
  Data Type Conversion28/1 -> Demux1/1
  in/1 -> Data Type Conversion28/1
  MatrixMultiply/1 -> out/1
  Constant1/1 -> MatrixMultiply/1
  Mux/1 -> MatrixMultiply/2
  Add1/1 -> Mux/2
  [cos_theta_el] -> Divide3/1
  Divide2/1 -> Add1/1
  [sin_theta_el] -> Divide2/1
  Divide3/1 -> Add1/2
  Demux1/1 -> Divide/2, Divide2/2  "i_d"
  Divide1/1 -> Add/2
  [cos_theta_el] -> Divide/1
  Divide/1 -> Add/1
  Add/1 -> Mux/1
  Demux1/2 -> Divide1/2, Divide3/2  "i_q"
  [sin_theta_el] -> Divide1/1
  Demux1/7 -> Mux/7
  Demux1/9 -> Mux/9
  Demux1/5 -> Mux/5
  Demux1/3 -> Mux/3
  Demux1/4 -> Mux/4
  Demux1/6 -> Mux/6
  Demux1/8 -> Mux/8

== system gm_Copy_of_uz_pmsm_model_9ph_21b_all_double_vnl/uz_pmsm_model_9ph/dq_model_9ph/Wrapped State DTI ==
  note: https://de.mathworks.com/help/releases/R2021a/hdlcoder/ug/troubleshoot-generate-implementation-model-from-simscape-pmsm.html?searchHighlight=troubleshoot-generate-implementation-model-from-simscape-pmsm&s_tid=doc_srchtitle
  Angular Speed : Inport
  polepair : Inport  Port=2
  reset : Inport  Port=3
  Compare To Constant : simulink/Logic and Bit Operations/Compare To Constant  relop=>=  const=single(pi)  OutDataTypeStr=boolean
  Compare To Constant1 : simulink/Logic and Bit Operations/Compare To Constant  relop=<  const=single(-pi)  OutDataTypeStr=boolean
  Constant : Constant  Value=double(2*pi)  SampleTime=-1
  Delay1 : Delay  DelayLength=1  ExternalReset=Level
      settings: InputPortMap=u0,r5
  Gain : Gain  Gain=ts
  Product : Product
  Sum : Sum  Inputs=|++
  Sum1 : Sum  Inputs=|-+
  Sum2 : Sum  Inputs=|++
  Switch : Switch  Criteria=u2 > Threshold  SaturateOnIntegerOverflow=off  InputSameDT=off
  Switch1 : Switch  Criteria=u2 > Threshold  SaturateOnIntegerOverflow=off  InputSameDT=off
  Angular Position : Outport
  wires:
  polepair/1 -> Product/2
  Angular Speed/1 -> Product/1
  Product/1 -> Gain/1
  reset/1 -> Delay1/2
  Gain/1 -> Sum/2
  Sum1/1 -> Switch/1
  Sum/1 -> Switch/3, Sum1/2, Compare To Constant/1
  Compare To Constant/1 -> Switch/2
  Switch/1 -> Switch1/3, Compare To Constant1/1, Sum2/2
  Switch1/1 -> Delay1/1  "Angular Position"
  Sum2/1 -> Switch1/1
  Constant/1 -> Sum1/1, Sum2/1
  Delay1/1 -> Angular Position/1, Sum/1
  Compare To Constant1/1 -> Switch1/2

== system gm_Copy_of_uz_pmsm_model_9ph_21b_all_double_vnl/uz_pmsm_model_9ph/dq_model_9ph/mechanical_system ==
  note: This delay breaks the algebraic loop between mechanical and electrical system.
      | Introduces a delay of 500ns.
  note: load torque negative!!!
  reset : Inport
  M_Mi : Inport  Port=2
  reciprocal_J : Inport  Port=3
  load_torque : Inport  Port=4
  Delay : Delay  DelayLength=1
  Product11 : Product
  Sum1 : Sum  Inputs=|++
  integrator : Subsystem
  omega_mech : Outport
  wires:
  reset/1 -> integrator/2(reset)
  Product11/1 -> integrator/1(in)
  integrator/1(outt) -> omega_mech/1
  Delay/1 -> Sum1/1
  M_Mi/1 -> Delay/1
  load_torque/1 -> Sum1/2
  Sum1/1 -> Product11/2
  reciprocal_J/1 -> Product11/1

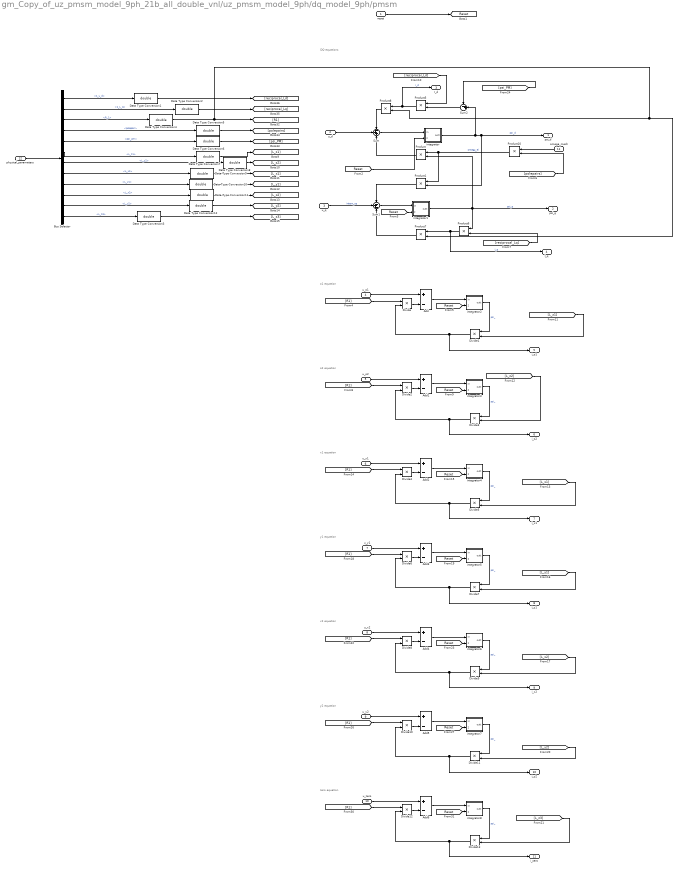
== system gm_Copy_of_uz_pmsm_model_9ph_21b_all_double_vnl/uz_pmsm_model_9ph/dq_model_9ph/pmsm ==
  note: zero equation
  note: y2 equation
  note: x2 equation
  note: y1 equation
  note: x1 equation
  note: o2 equation
  note: DQ equations
  note: o1 equation
  reset : Inport
  u_d : Inport  Port=2
  u_q : Inport  Port=3
  u_o1 : Inport  Port=4
  u_o2 : Inport  Port=5
  u_x1 : Inport  Port=6
  u_y1 : Inport  Port=7
  u_x2 : Inport  Port=8
  u_y2 : Inport  Port=9
  u_zero : Inport  Port=10
  omega_mech : Inport  Port=11
  physical_parameters : Inport  Port=12
  Add{,1..6} (7 alike) : Sum  Inputs=+-
  Bus Selector : BusSelector  OutputSignals=1_L_d,1_L_q,R_1,polepair,psi_pm,L_z1,L_z2,L_x1,L_y1,L_x2,L_y2,L_z3
  Data Type Conversion{1..12} (12 alike) : DataTypeConversion  OutDataTypeStr=double  RndMeth=Nearest  SaturateOnIntegerOverflow=off
  Divide{,1..13} (14 alike) : Product  Inputs=**
  Product{,1,5..8,10} (7 alike) : Product
  Sum : Sum  Inputs=-++
  Sum1 : Sum  Inputs=-+-
  Sum2 : Sum  Inputs=-+|
  integrator : Subsystem
  integrator1 : Subsystem
  integrator2 : Subsystem
  integrator3 : Subsystem
  integrator4 : Subsystem
  integrator5 : Subsystem
  integrator6 : Subsystem
  integrator7 : Subsystem
  integrator8 : Subsystem
  psi_d : Outport
  psi_q : Outport  Port=2
  I_d : Outport  Port=3
  I_q : Outport  Port=4
  i_o1 : Outport  Port=5
  i_o2 : Outport  Port=6
  i_x1 : Outport  Port=7
  i_y1 : Outport  Port=8
  i_x2 : Outport  Port=9
  i_y2 : Outport  Port=10
  i_zero : Outport  Port=11
  tag scope: Reset=global
  wires:
  Data Type Conversion12/1 -> [L_y2]
  Data Type Conversion11/1 -> [L_x2]
  Data Type Conversion10/1 -> [L_y1]
  Data Type Conversion9/1 -> [L_x1]
  Data Type Conversion8/1 -> [L_z2]
  Data Type Conversion7/1 -> [L_z1]
  Data Type Conversion6/1 -> [psi_PM]
  Data Type Conversion5/1 -> [polepairs]
  Data Type Conversion4/1 -> Product8/2, Product7/2, [R1]
  Data Type Conversion2/1 -> [reciprocal_Lq]
  Bus Selector/12 -> Data Type Conversion3/1  "<L_z3>"
  Data Type Conversion3/1 -> [L_z3]
  Data Type Conversion1/1 -> [reciprocal_Ld]
  u_d/1 -> Sum/2
  Add6/1 -> integrator8/1(in)
  Add5/1 -> integrator7/1(in)
  Add4/1 -> integrator6/1(in)
  Add3/1 -> integrator5/1(in)
  Add2/1 -> integrator4/1(in)
  Add1/1 -> integrator3/1(in)
  Add/1 -> integrator2/1(in)
  Sum1/1 -> integrator1/1(in)
  Sum/1 -> integrator/1(in)
  [L_z3] -> Divide13/2
  [L_y2] -> Divide11/2
  [L_x2] -> Divide9/2
  [L_y1] -> Divide7/2
  [L_x1] -> Divide5/2
  [polepairs] -> Product10/2
  Bus Selector/9 -> Data Type Conversion10/1  "<L_y1>"
  physical_parameters/1 -> Bus Selector/1
  Bus Selector/10 -> Data Type Conversion11/1  "<L_x2>"
  Bus Selector/3 -> Data Type Conversion4/1  "<R_1>"
  Bus Selector/11 -> Data Type Conversion12/1  "<L_y2>"
  Bus Selector/7 -> Data Type Conversion8/1  "<L_z2>"
  Bus Selector/6 -> Data Type Conversion7/1  "<L_z1>"
  Bus Selector/5 -> Data Type Conversion6/1  "<psi_pm>"
  Bus Selector/2 -> Data Type Conversion2/1  "<1_L_q>"
  Bus Selector/8 -> Data Type Conversion9/1  "<L_x1>"
  Bus Selector/4 -> Data Type Conversion5/1  "<polepair>"
  Bus Selector/1 -> Data Type Conversion1/1  "<1_L_d>"
  integrator8/1(outt) -> Divide13/1  "psi_"
  [R1] -> Divide12/1
  Divide12/1 -> Add6/2
  Divide13/1 -> Divide12/2, i_zero/1
  u_zero/1 -> Add6/1
  [Reset] -> integrator8/2(reset)
  [Reset] -> integrator7/2(reset)
  u_y2/1 -> Add5/1
  Divide11/1 -> Divide10/2, i_y2/1
  Divide10/1 -> Add5/2
  [R1] -> Divide10/1
  integrator7/1(outt) -> Divide11/1  "psi_"
  integrator6/1(outt) -> Divide9/1  "psi_"
  [R1] -> Divide8/1
  Divide8/1 -> Add4/2
  Divide9/1 -> Divide8/2, i_x2/1
  u_x2/1 -> Add4/1
  [Reset] -> integrator6/2(reset)
  [Reset] -> integrator5/2(reset)
  u_y1/1 -> Add3/1
  Divide7/1 -> Divide6/2, i_y1/1
  Divide6/1 -> Add3/2
  [R1] -> Divide6/1
  integrator5/1(outt) -> Divide7/1  "psi_"
  integrator4/1(outt) -> Divide5/1  "psi_"
  [R1] -> Divide4/1
  Divide4/1 -> Add2/2
  Divide5/1 -> Divide4/2, i_x1/1
  u_x1/1 -> Add2/1
  [Reset] -> integrator4/2(reset)
  [Reset] -> integrator3/2(reset)
  [L_z2] -> Divide3/2
  u_o2/1 -> Add1/1
  Divide3/1 -> Divide2/2, i_o2/1
  Divide2/1 -> Add1/2
  [R1] -> Divide2/1
  integrator3/1(outt) -> Divide3/1  "psi_"
  integrator2/1(outt) -> Divide1/1  "psi_"
  [R1] -> Divide/1
  Divide/1 -> Add/2
  Divide1/1 -> Divide/2, i_o1/1
  u_o1/1 -> Add/1
  [L_z1] -> Divide1/2
  [Reset] -> integrator2/2(reset)
  [Reset] -> integrator1/2(reset)
  [Reset] -> integrator/2(reset)
  reset/1 -> [Reset]
  Product7/1 -> Sum1/3
  [reciprocal_Lq] -> Product6/2
  Product8/1 -> Sum/1
  Sum2/1 -> Product5/2
  integrator/1(outt) -> Product1/2, psi_d/1, Sum2/2  "psi_d"
  Product10/1 -> Product/1, Product1/1  "omega_el"
  Product6/1 -> Product7/1, I_q/1  "I_q"
  [psi_PM] -> Sum2/1
  Product1/1 -> Sum1/1
  integrator1/1(outt) -> Product6/1, Product/2, psi_q/1  "psi_q"
  [reciprocal_Ld] -> Product5/1
  Product5/1 -> Product8/1, I_d/1  "I_d"
  Product/1 -> Sum/3
  u_q/1 -> Sum1/2  "intern_uq"
  omega_mech/1 -> Product10/1

== system gm_Copy_of_uz_pmsm_model_9ph_21b_all_double_vnl/uz_pmsm_model_9ph/dq_model_9ph/torque_calculation ==
  I_d : Inport
  I_q : Inport  Port=2
  psi_d : Inport  Port=3
  psi_q : Inport  Port=4
  polepairs : Inport  Port=5
  Factor : Gain  Gain=9/2
  Product2 : Product
  Product3 : Product
  Product9 : Product
  Sum3 : Sum  Inputs=-|+
  M_Mi : Outport
  wires:
  Factor/1 -> Product9/1  "M_Mi"
  polepairs/1 -> Product9/2
  Product9/1 -> M_Mi/1  "M_Mi"
  I_q/1 -> Product3/2
  I_d/1 -> Product2/1
  psi_d/1 -> Product3/1
  psi_q/1 -> Product2/2
  Product2/1 -> Sum3/1
  Product3/1 -> Sum3/2
  Sum3/1 -> Factor/1

== system gm_Copy_of_uz_pmsm_model_9ph_21b_all_double_vnl/uz_pmsm_model_9ph/abc_to_dq_vnl/Line-Line to Phase voltage/abc   to   alpha_beta_0 ==
  "a, b, c" : Inport  PortDimensions=3
  Gain2 : Gain  Gain=2/3  ParamDataTypeStr=fixdt(1,18,16)  SaturateOnIntegerOverflow=on  OutDataTypeStr=Inherit: Same as input
  Gain4 : Gain  Gain="[ 1   -0.5   -0.5; 0   0.5*sqrt(3)   -0.5*sqrt(3); 0.5  0.5  0.5 ]"  Multiplication=Matrix(K*u) (u vector)  ParamDataTypeStr=fixdt(1,18,16)  OutDataTypeStr=fixdt(1,25,12)  SaturateOnIntegerOverflow=on
  "alpha, beta, 0 " : Outport
  wires:
  Gain4/1 -> Gain2/1
  "a, b, c"/1 -> Gain4/1
  Gain2/1 -> "alpha, beta, 0 "/1

== system gm_Copy_of_uz_pmsm_model_9ph_21b_all_double_vnl/uz_pmsm_model_9ph/abc_to_dq_vnl/Line-Line to Phase voltage/alpha_beta_0   to   abc ==
  "alpha, beta, 0  " : Inport  PortDimensions=3
  Gain4 : Gain  Gain="[ 1 0 1; -0.5   0.5*sqrt(3)  1; -0.5 -0.5*sqrt(3) 1 ]"  Multiplication=Matrix(K*u) (u vector)  ParamDataTypeStr=fixdt(1,18,16)  SaturateOnIntegerOverflow=on  OutDataTypeStr=Inherit: Same as input
  "a, b, c" : Outport
  wires:
  "alpha, beta, 0  "/1 -> Gain4/1
  Gain4/1 -> "a, b, c"/1

== system gm_Copy_of_uz_pmsm_model_9ph_21b_all_double_vnl/uz_pmsm_model_9ph/abc_to_dq_vnl/Line-Line to Phase voltage1/abc   to   alpha_beta_0 ==
  "a, b, c" : Inport  PortDimensions=3
  Gain2 : Gain  Gain=2/3  ParamDataTypeStr=fixdt(1,18,16)  SaturateOnIntegerOverflow=on  OutDataTypeStr=Inherit: Same as input
  Gain4 : Gain  Gain="[ 1   -0.5   -0.5; 0   0.5*sqrt(3)   -0.5*sqrt(3); 0.5  0.5  0.5 ]"  Multiplication=Matrix(K*u) (u vector)  ParamDataTypeStr=fixdt(1,18,16)  OutDataTypeStr=fixdt(1,25,12)  SaturateOnIntegerOverflow=on
  "alpha, beta, 0 " : Outport
  wires:
  Gain2/1 -> "alpha, beta, 0 "/1
  "a, b, c"/1 -> Gain4/1
  Gain4/1 -> Gain2/1

== system gm_Copy_of_uz_pmsm_model_9ph_21b_all_double_vnl/uz_pmsm_model_9ph/abc_to_dq_vnl/Line-Line to Phase voltage1/alpha_beta_0   to   abc ==
  "alpha, beta, 0  " : Inport  PortDimensions=3
  Gain4 : Gain  Gain="[ 1 0 1; -0.5   0.5*sqrt(3)  1; -0.5 -0.5*sqrt(3) 1 ]"  Multiplication=Matrix(K*u) (u vector)  ParamDataTypeStr=fixdt(1,18,16)  SaturateOnIntegerOverflow=on  OutDataTypeStr=Inherit: Same as input
  "a, b, c" : Outport
  wires:
  Gain4/1 -> "a, b, c"/1
  "alpha, beta, 0  "/1 -> Gain4/1
